simulink subsystem "MLI_20_layer_pipe"  (R2024b)
settings: Solver=VariableStepAuto  StartTime=0.0  StopTime=10.0  RelTol=1e-3
settings Model: Creator=MW  LastModifiedBy=MW

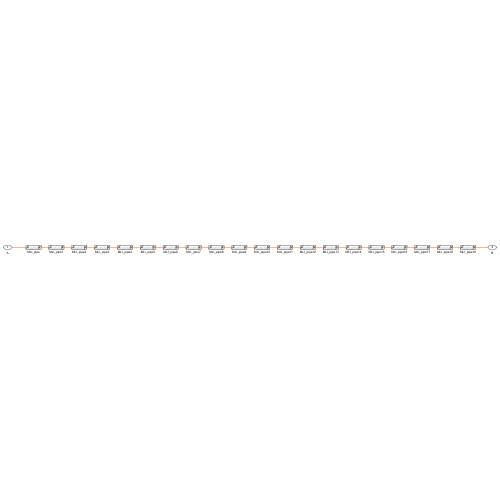
[thumbnail: Simulink's stored preview of the top-level diagram]
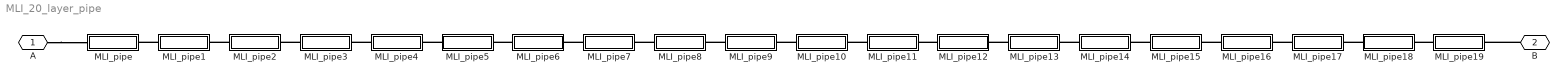
== system MLI_20_layer_pipe ==
  MLI_pipe{,1..19} (20 alike) : Subsystem  ReferencedSubsystem=MIL_1_layer_radiative_pipe
      settings: PortSchema="{\"entries\":[{\"content\":{\"sides\":[{\"content\":{\"connectorIds\":[\"LConn1\"]},\"type\":\"ConnectorPlacement.EquallySpacedRectSide\",\"uuid\":\"13959ff0-7161-4264-b74c-d5f6fc1fc79f\"},{\"content\":{\"connectorIds\":[\"LConn2\"],\"side\":\"RIGHT\"},\"type\":\"ConnectorPlacement.EquallySpacedRectSide\",\"uuid\":\"0144929d-c826-44a3-abc2-3c69c72d534c\"},{\"content\":{\"side\":\"TOP\"},\"type\":\"ConnectorPlacement.EquallySpacedRectSide\",\"uuid\":\"bda55155-c7f6-4e1e-b7ae-8f65907cbe02\"}]},\"type\":\"ConnectorPlacement.EquallySpacedConnector\",\"uuid\":\"e24db636-ea4a-4050-86a0-b249fb595212\"}],\"packageUris\":[\"http://schema.mathworks.com/mf0/Connector/R2020b\"],\"version\":\"1.0\"}"
  A : PMIOPort  Side=Left
  B : PMIOPort  Port=2  Side=Left
  connections:
  MLI_pipe1/LConn1 -- MLI_pipe/LConn2
  A/RConn1 -- MLI_pipe/LConn1
  MLI_pipe3/LConn1 -- MLI_pipe2/LConn2
  MLI_pipe2/LConn1 -- MLI_pipe1/LConn2
  MLI_pipe4/LConn1 -- MLI_pipe3/LConn2
  MLI_pipe7/LConn1 -- MLI_pipe6/LConn2
  MLI_pipe6/LConn1 -- MLI_pipe5/LConn2
  MLI_pipe8/LConn1 -- MLI_pipe7/LConn2
  MLI_pipe9/LConn1 -- MLI_pipe8/LConn2
  MLI_pipe5/LConn1 -- MLI_pipe4/LConn2
  MLI_pipe14/LConn1 -- MLI_pipe13/LConn2
  MLI_pipe19/LConn1 -- MLI_pipe18/LConn2
  MLI_pipe17/LConn1 -- MLI_pipe16/LConn2
  MLI_pipe15/LConn1 -- MLI_pipe14/LConn2
  MLI_pipe18/LConn1 -- MLI_pipe17/LConn2
  MLI_pipe12/LConn1 -- MLI_pipe11/LConn2
  MLI_pipe11/LConn1 -- MLI_pipe10/LConn2
  MLI_pipe16/LConn1 -- MLI_pipe15/LConn2
  MLI_pipe13/LConn1 -- MLI_pipe12/LConn2
  MLI_pipe10/LConn1 -- MLI_pipe9/LConn2
  B/RConn1 -- MLI_pipe19/LConn2
